simulink model "OpenLoopTest_asesoria"  (R2023a)
settings: Solver=VariableStepAuto  StartTime=0.0  StopTime=30  RelTol=1e-3
undefined symbols (not defined in the file): B, Iw, Ke, Kt, La, Ra
libraries: simulink_extras x3
settings Model: Creator=Personal  LastModifiedBy=informatica
settings OptimizationCC: ReuseModelBlockBuffer=off

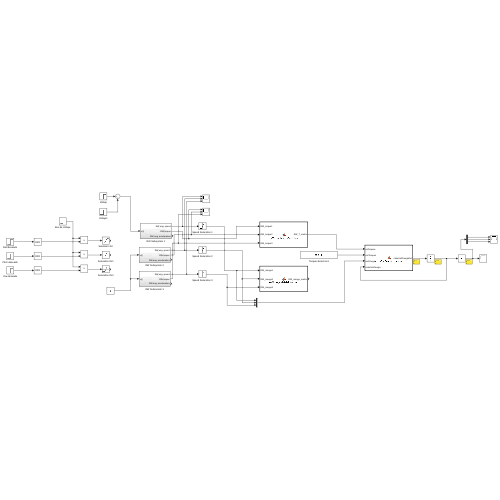
[thumbnail: Simulink's stored preview of the top-level diagram]
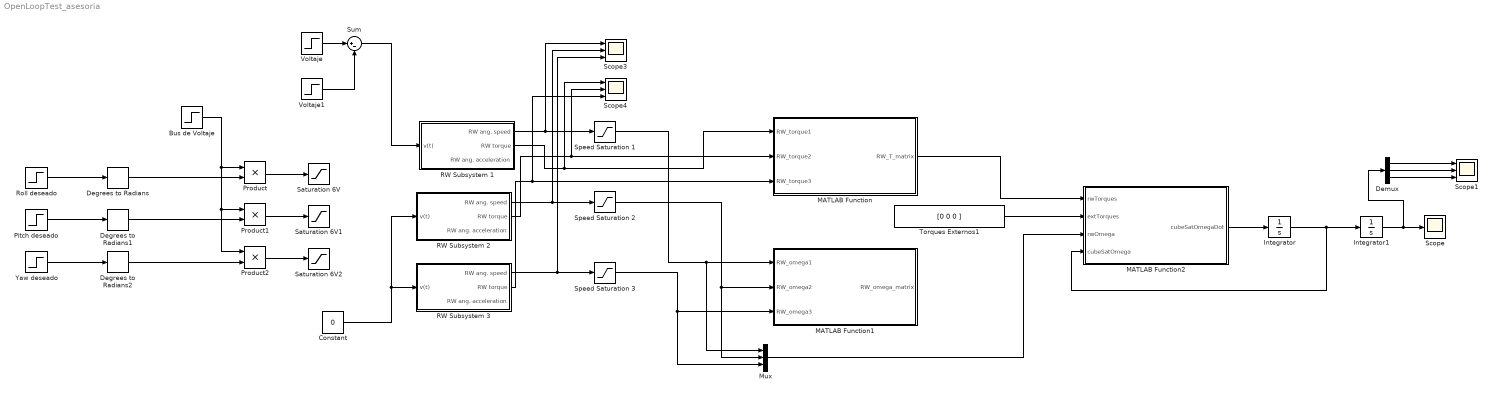
== system OpenLoopTest_asesoria ==
  Bus de Voltaje : Step  Time=2  After=12  SampleTime=0
  Constant : Constant  Value=0
  Degrees to Radians : simulink_extras/Transformations/Degrees to Radians
  Degrees to Radians1 : simulink_extras/Transformations/Degrees to Radians
  Degrees to Radians2 : simulink_extras/Transformations/Degrees to Radians
  Demux : Demux  Outputs=3
  Integrator : Integrator  InitialCondition=[0 0 0]
  Integrator1 : Integrator  InitialCondition=[0 0 0]
  MATLAB Function : MATLAB Function  TreatAsAtomicUnit=on
  MATLAB Function1 : MATLAB Function  TreatAsAtomicUnit=on
  MATLAB Function2 : MATLAB Function  TreatAsAtomicUnit=on
  Mux : Mux  Inputs=3
  Pitch deseado : Step  Time=2  After=0  SampleTime=0
  Product : Product
  Product1 : Product
  Product2 : Product
  RW Subsystem 1 : Subsystem
  RW Subsystem 2 : Subsystem
  RW Subsystem 3 : Subsystem
  Roll deseado : Step  Time=2  After=90  SampleTime=0
  Saturation 6V : Saturate  UpperLimit=6  LowerLimit=0
  Saturation 6V1 : Saturate  UpperLimit=6  LowerLimit=0
  Saturation 6V2 : Saturate  UpperLimit=6  LowerLimit=0
  Scope : Scope
  Scope1 : Scope  NumInputPorts=3
  Scope3 : Scope  NumInputPorts=3
  Scope4 : Scope  NumInputPorts=3
  Speed Saturation 1 : Saturate  UpperLimit=8000  LowerLimit=-8000
  Speed Saturation 2 : Saturate  UpperLimit=8000  LowerLimit=0
  Speed Saturation 3 : Saturate  UpperLimit=8000  LowerLimit=0
  Sum : Sum  Inputs=|+-
  Torques Externos1 : Constant  Value=[0 0 0 ]
  Voltaje : Step  Time=2  After=3  SampleTime=0
  Voltaje1 : Step  Time=10  After=6  SampleTime=0
  Yaw deseado : Step  Time=2  After=180  SampleTime=0
  wires:
  Roll deseado/1 -> Degrees to Radians/1
  Yaw deseado/1 -> Degrees to Radians2/1
  Pitch deseado/1 -> Degrees to Radians1/1
  Bus de Voltaje/1 -> Product2/1, Product1/1, Product/1
  Degrees to Radians/1 -> Product/2
  Degrees to Radians1/1 -> Product1/2
  Degrees to Radians2/1 -> Product2/2
  Product/1 -> Saturation 6V/1
  Product1/1 -> Saturation 6V1/1
  Product2/1 -> Saturation 6V2/1
  RW Subsystem 1/1(RW ang. speed) -> Scope3/1, Speed Saturation 1/1
  RW Subsystem 2/1(RW ang. speed) -> Scope3/2, Speed Saturation 2/1
  RW Subsystem 3/1(RW ang. speed) -> Scope3/3, Speed Saturation 3/1
  RW Subsystem 1/2(RW torque) -> Scope4/1, MATLAB Function/1(RW_torque1)
  RW Subsystem 2/2(RW torque) -> Scope4/2, MATLAB Function/2(RW_torque2)
  RW Subsystem 3/2(RW torque) -> Scope4/3, MATLAB Function/3(RW_torque3)
  Speed Saturation 1/1 -> Mux/1, MATLAB Function1/1(RW_omega1)
  Speed Saturation 2/1 -> Mux/2, MATLAB Function1/2(RW_omega2)
  Speed Saturation 3/1 -> Mux/3, MATLAB Function1/3(RW_omega3)
  MATLAB Function/1(RW_T_matrix) -> MATLAB Function2/1(rwTorques)
  MATLAB Function2/1(cubeSatOmegaDot) -> Integrator/1
  Integrator/1 -> MATLAB Function2/4(cubeSatOmega), Integrator1/1
  Integrator1/1 -> Demux/1, Scope/1
  Torques Externos1/1 -> MATLAB Function2/2(extTorques)
  Constant/1 -> RW Subsystem 2/1(v(t)), RW Subsystem 3/1(v(t))
  Mux/1 -> MATLAB Function2/3(rwOmega)
  Demux/1 -> Scope1/1
  Demux/2 -> Scope1/2
  Demux/3 -> Scope1/3
  Voltaje/1 -> Sum/1
  Sum/1 -> RW Subsystem 1/1(v(t))
  Voltaje1/1 -> Sum/2

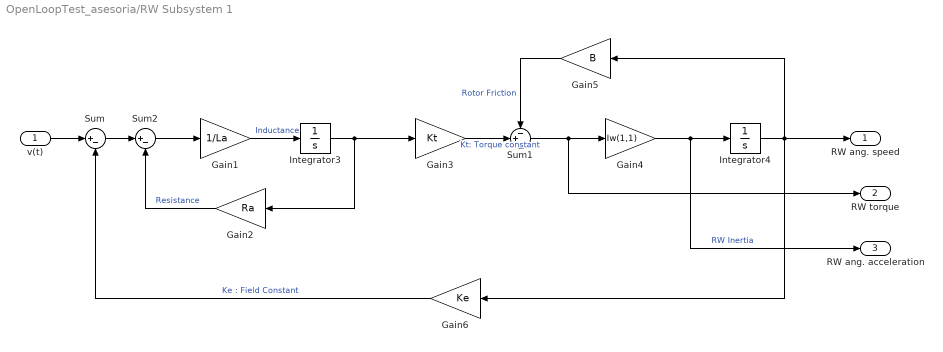
== system OpenLoopTest_asesoria/RW Subsystem 1 ==
  v(t) : Inport
  Gain1 : Gain  Gain=1/La
  Gain2 : Gain  Gain=Ra
  Gain3 : Gain  Gain=Kt
  Gain4 : Gain  Gain=Iw(1,1)
  Gain5 : Gain  Gain=B
  Gain6 : Gain  Gain=Ke
  Integrator3 : Integrator
  Integrator4 : Integrator
  Sum : Sum  Inputs=|+-
  Sum1 : Sum  Inputs=-+|
  Sum2 : Sum  Inputs=|+-
  RW ang. speed : Outport  VectorParamsAs1DForOutWhenUnconnected=off
  RW torque : Outport  Port=2  VectorParamsAs1DForOutWhenUnconnected=off
  RW ang. acceleration : Outport  Port=3  VectorParamsAs1DForOutWhenUnconnected=off
  wires:
  Gain2/1 -> Sum2/2  "Resistance"
  Integrator3/1 -> Gain2/1, Gain3/1
  Gain6/1 -> Sum/2  "Ke : Field Constant"
  Gain5/1 -> Sum1/1  "Rotor Friction"
  v(t)/1 -> Sum/1
  Sum2/1 -> Gain1/1
  Sum1/1 -> Gain4/1, RW torque/1
  Integrator4/1 -> Gain5/1, Gain6/1, RW ang. speed/1
  Gain4/1 -> Integrator4/1, RW ang. acceleration/1  "RW Inertia"
  Gain1/1 -> Integrator3/1  "Inductance"
  Gain3/1 -> Sum1/2  "Kt: Torque constant"
  Sum/1 -> Sum2/1

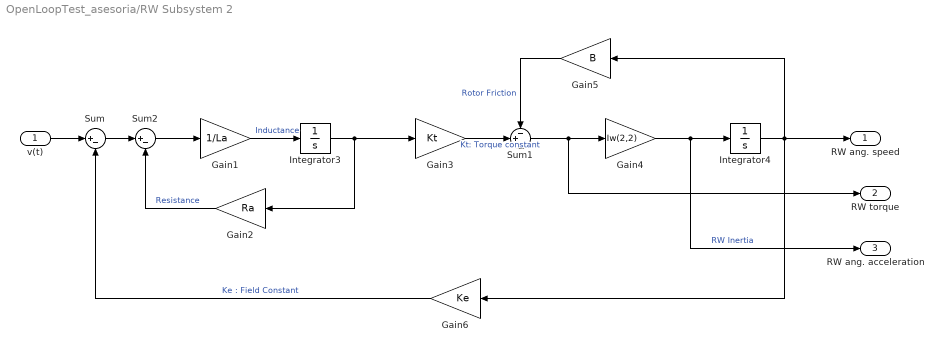
== system OpenLoopTest_asesoria/RW Subsystem 2 ==
  v(t) : Inport
  Gain1 : Gain  Gain=1/La
  Gain2 : Gain  Gain=Ra
  Gain3 : Gain  Gain=Kt
  Gain4 : Gain  Gain=Iw(2,2)
  Gain5 : Gain  Gain=B
  Gain6 : Gain  Gain=Ke
  Integrator3 : Integrator
  Integrator4 : Integrator
  Sum : Sum  Inputs=|+-
  Sum1 : Sum  Inputs=-+|
  Sum2 : Sum  Inputs=|+-
  RW ang. speed : Outport  VectorParamsAs1DForOutWhenUnconnected=off
  RW torque : Outport  Port=2  VectorParamsAs1DForOutWhenUnconnected=off
  RW ang. acceleration : Outport  Port=3  VectorParamsAs1DForOutWhenUnconnected=off
  wires:
  Sum/1 -> Sum2/1
  Gain3/1 -> Sum1/2  "Kt: Torque constant"
  Gain1/1 -> Integrator3/1  "Inductance"
  Gain4/1 -> RW ang. acceleration/1, Integrator4/1  "RW Inertia"
  Integrator4/1 -> RW ang. speed/1, Gain6/1, Gain5/1
  Sum1/1 -> RW torque/1, Gain4/1
  Sum2/1 -> Gain1/1
  v(t)/1 -> Sum/1
  Gain5/1 -> Sum1/1  "Rotor Friction"
  Gain6/1 -> Sum/2  "Ke : Field Constant"
  Integrator3/1 -> Gain3/1, Gain2/1
  Gain2/1 -> Sum2/2  "Resistance"

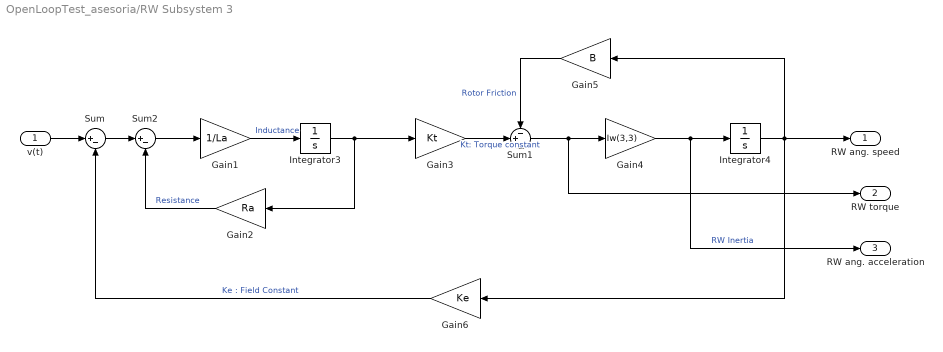
== system OpenLoopTest_asesoria/RW Subsystem 3 ==
  v(t) : Inport
  Gain1 : Gain  Gain=1/La
  Gain2 : Gain  Gain=Ra
  Gain3 : Gain  Gain=Kt
  Gain4 : Gain  Gain=Iw(3,3)
  Gain5 : Gain  Gain=B
  Gain6 : Gain  Gain=Ke
  Integrator3 : Integrator
  Integrator4 : Integrator
  Sum : Sum  Inputs=|+-
  Sum1 : Sum  Inputs=-+|
  Sum2 : Sum  Inputs=|+-
  RW ang. speed : Outport  VectorParamsAs1DForOutWhenUnconnected=off
  RW torque : Outport  Port=2  VectorParamsAs1DForOutWhenUnconnected=off
  RW ang. acceleration : Outport  Port=3  VectorParamsAs1DForOutWhenUnconnected=off
  wires:
  Gain2/1 -> Sum2/2  "Resistance"
  Integrator3/1 -> Gain2/1, Gain3/1
  Gain6/1 -> Sum/2  "Ke : Field Constant"
  Gain5/1 -> Sum1/1  "Rotor Friction"
  v(t)/1 -> Sum/1
  Sum2/1 -> Gain1/1
  Sum1/1 -> Gain4/1, RW torque/1
  Integrator4/1 -> Gain5/1, Gain6/1, RW ang. speed/1
  Gain4/1 -> Integrator4/1, RW ang. acceleration/1  "RW Inertia"
  Gain1/1 -> Integrator3/1  "Inductance"
  Gain3/1 -> Sum1/2  "Kt: Torque constant"
  Sum/1 -> Sum2/1

== matlab function OpenLoopTest_asesoria/MATLAB Function1 ==
  data: RW_omega1 input; RW_omega_matrix output; RW_omega2 input; RW_omega3 input
function RW_omega_matrix = rwOmegaMatrixFunction(RW_omega1,RW_omega2,RW_omega3)
%#codegen

RW_omega_matrix = [RW_omega1;
                   RW_omega2;
                   RW_omega3];

== matlab function OpenLoopTest_asesoria/MATLAB Function ==
  data: RW_torque1 input; RW_T_matrix output; RW_torque2 input; RW_torque3 input
function RW_T_matrix = rwTorqueMatrixFunction(RW_torque1,RW_torque2,RW_torque3)
%#codegen

RW_T_matrix = [RW_torque1;
               RW_torque2;
               RW_torque3];

== matlab function OpenLoopTest_asesoria/MATLAB Function2 ==
  data: rwTorques input; cubeSatOmegaDot output; extTorques input; rwOmega input; cubeSatOmega input
function cubeSatOmegaDot = cubeSatDynamicModel(rwTorques,extTorques,rwOmega,cubeSatOmega)

% Inercia EyasSat [kg m2]
I =(4*0.3^2/6)*[1 0 0 ; 0 1 0; 0 0 1];

%Momentos de inercia EyasSat
Ixx = I(1,1);
Iyy = I(2,2);
Izz = I(3,3);

% Inercia EyasSat [kg m2]
Iw = 3e-6*[1 0 0 ; 0 1 0; 0 0 1]; %kg m2

%Momento angular RW
hw = Iw*rwOmega;

%Velocidades angulares EyasSat
wx = cubeSatOmega(1);
wy = cubeSatOmega(2);
wz = cubeSatOmega(3);

%Torques externos
Tx = extTorques(1);
Ty = extTorques(2);
Tz = extTorques(3);

%Torques de control
Tc_x = rwTorques(1);
Tc_y = rwTorques(2);
Tc_z = rwTorques(3);

hx = hw(1);
hy = hw(2);
hz = hw(3);

omegaDotX = (Tx+Tc_x+wy*wz*(Iyy-Izz)-hz*wy+hy*wz)/Ixx;
omegaDotY = (Ty+Tc_y+wx*wz*(Izz-Ixx)-hx*wz+hz*wx)/Iyy;
omegaDotZ = (Tz+Tc_z+wx*wy*(Ixx-Iyy)-hy*wx+hx*wy)/Izz;

cubeSatOmegaDot = [omegaDotX omegaDotY omegaDotZ];
